simulink model "host"  (R2019a)
settings: Solver=VariableStepAuto  StartTime=0.0  StopTime=inf  RelTol=1e-3  EnableMultiTasking=on
undefined symbols (not defined in the file): f
libraries: instrumentlib x8
settings Model: ExtModeTrigDuration=2  Creator=Duc  LastModifiedBy=Mustafa
settings SolverCC: PositivePriorityOrder=on
settings OptimizationCC: EnhancedBackFolding=on  PassReuseOutputArgsAs=Individual arguments  ZeroExternalMemoryAtStartup=off  ZeroInternalMemoryAtStartup=off  MaxStackSize=64  OptimizeBlockOrder=speed  DifferentSizesBufferReuse=on  OptimizationCustomize=off
settings DebuggingCC: ParameterTunabilityLossMsg=error
settings HardwareCC: ProdBitPerPointer=32  ProdBitPerSizeT=32  ProdBitPerPtrDiffT=32  ProdLargestAtomicInteger=Long  ProdWordSize=32  ProdHWDeviceType=ARM Compatible->ARM 9  UseEmbeddedCoderFeatures=off  UseSimulinkCoderFeatures=off
settings SFSimCC: MATLABDynamicMemAlloc=off
settings RTWCC: SystemTargetFile=ert.tlc  HardwareBoard=LEGO MINDSTORMS EV3  TLCOptions="-aInlineSetEventsForThisBaseRateFcn=TLC_FALSE -aSuppressMultiTaskScheduler=TLC_FALSE  -aRateBasedStepFcn=0"  TemplateMakefile=ert_default_tmf  GenerateReport=on  Toolchain=Sourcery G++ Lite v2009q3  IncludeHyperlinkInReport=on  LaunchReport=on  GenerateTraceInfo=on  GenerateTraceReport=on  GenerateTraceReportSl=on  GenerateTraceReportSf=on  GenerateTraceReportEml=on
settings CodeAppCC: ForceParamTrailComments=on  IgnoreCustomStorageClasses=off  OperatorAnnotations=on  SimulinkDataObjDesc=on  SFDataObjDesc=on  InsertBlockDesc=on
settings ERTTargetCC: SupportContinuousTime=on  SupportNonInlinedSFcns=on  SupportVariableSizeSignals=on

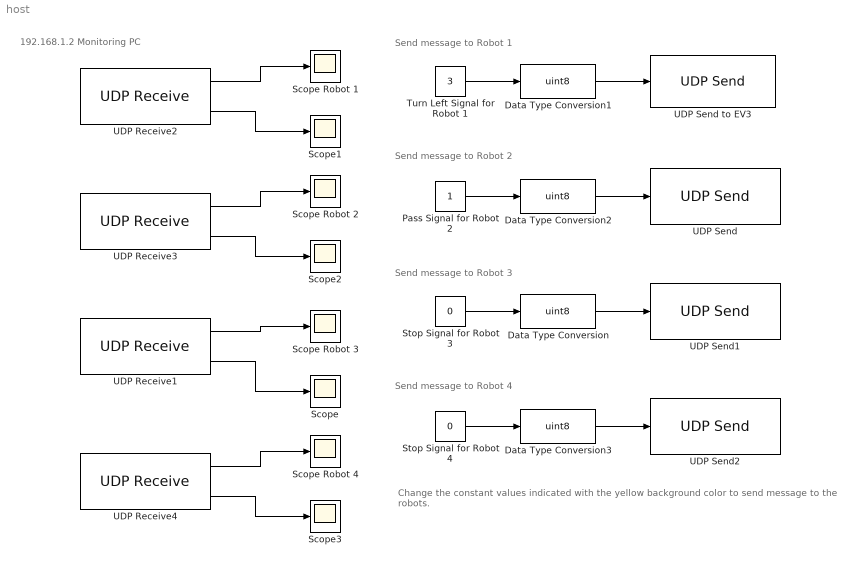
== system host ==
  note: Change the constant values indicated
      | with the yellow background color
      | to send message to the robots.
  note: Send message to Robot 1
  note: 192.168.1.2 Monitoring PC
  note: Send message to Robot 2
  note: Send message to Robot 3
  note: Send message to Robot 4
  Data Type Conversion{,1..3} (4 alike) : DataTypeConversion  OutDataTypeStr=uint8
  Pass Signal for Robot 2 : Constant
  Scope{,1..3} (4 alike) : Scope
  Scope Robot {1..4} (4 alike) : Scope
  Stop Signal for Robot 3 : Constant  Value=0
  Stop Signal for Robot 4 : Constant  Value=0
  Turn Left Signal for Robot 1 : Constant  Value=3
  UDP Receive1 : instrumentlib/UDP Receive  Host=localhost  Port=9090  LocalPort=25003  EnablePortSharing=off  GetLatestData=off  DataSize=[1 1]  DataType=uint8  ASCIIFormatting=%f,  Terminator=LF  ByteOrder=BigEndian  EnableBlockingMode=off  Timeout=10  SampleTime=1  LocalAddress=192.168.1.2
      settings: SourceProductName=Instrument Control Toolbox
  UDP Receive2 : instrumentlib/UDP Receive  Host=localhost  Port=9090  LocalPort=25001  EnablePortSharing=off  GetLatestData=off  DataSize=[1 1]  DataType=uint8  ASCIIFormatting=%f,  Terminator=LF  ByteOrder=BigEndian  EnableBlockingMode=off  Timeout=10  SampleTime=1  LocalAddress=192.168.1.2
      settings: SourceProductName=Instrument Control Toolbox
  UDP Receive3 : instrumentlib/UDP Receive  Host=localhost  Port=9090  LocalPort=25002  EnablePortSharing=off  GetLatestData=off  DataSize=[1 1]  DataType=uint8  ASCIIFormatting=%f,  Terminator=LF  ByteOrder=BigEndian  EnableBlockingMode=off  Timeout=10  SampleTime=1  LocalAddress=192.168.1.2
      settings: SourceProductName=Instrument Control Toolbox
  UDP Receive4 : instrumentlib/UDP Receive  Host=localhost  Port=9090  LocalPort=25004  EnablePortSharing=off  GetLatestData=off  DataSize=[1 1]  DataType=uint8  ASCIIFormatting=%f,  Terminator=LF  ByteOrder=BigEndian  EnableBlockingMode=off  Timeout=10  SampleTime=1  LocalAddress=192.168.1.2
      settings: SourceProductName=Instrument Control Toolbox
  UDP Send : instrumentlib/UDP Send  Host=192.168.1.3  Port=25000  LocalPort=-1  EnablePortSharing=off  ByteOrder=BigEndian  OutputDatagramPacketSize=512  EnableBlockingMode=on  LocalAddress=0.0.0.0
      settings: SourceProductName=Instrument Control Toolbox
  UDP Send to EV3 : instrumentlib/UDP Send  Host=192.168.1.4  Port=25000  LocalPort=-1  EnablePortSharing=off  ByteOrder=LittleEndian  OutputDatagramPacketSize=512  EnableBlockingMode=on  LocalAddress=0.0.0.0
      settings: SourceProductName=Instrument Control Toolbox
  UDP Send1 : instrumentlib/UDP Send  Host=192.168.1.6  Port=25000  LocalPort=-1  EnablePortSharing=off  ByteOrder=BigEndian  OutputDatagramPacketSize=512  EnableBlockingMode=on  LocalAddress=0.0.0.0
      settings: SourceProductName=Instrument Control Toolbox
  UDP Send2 : instrumentlib/UDP Send  Host=192.168.1.9  Port=25000  LocalPort=-1  EnablePortSharing=off  ByteOrder=BigEndian  OutputDatagramPacketSize=512  EnableBlockingMode=on  LocalAddress=0.0.0.0
      settings: SourceProductName=Instrument Control Toolbox
  wires:
  UDP Receive1/1 -> Scope Robot 3/1
  Data Type Conversion2/1 -> UDP Send/1
  Stop Signal for Robot 3/1 -> Data Type Conversion/1
  Data Type Conversion3/1 -> UDP Send2/1
  Data Type Conversion/1 -> UDP Send1/1
  UDP Receive1/2 -> Scope/1
  UDP Receive2/1 -> Scope Robot 1/1
  UDP Receive2/2 -> Scope1/1
  UDP Receive3/1 -> Scope Robot 2/1
  UDP Receive3/2 -> Scope2/1
  UDP Receive4/1 -> Scope Robot 4/1
  UDP Receive4/2 -> Scope3/1
  Turn Left Signal for Robot 1/1 -> Data Type Conversion1/1
  Data Type Conversion1/1 -> UDP Send to EV3/1
  Pass Signal for Robot 2/1 -> Data Type Conversion2/1
  Stop Signal for Robot 4/1 -> Data Type Conversion3/1
